simulink model "adc"  (R2017a)
settings: Solver=VariableStepAuto  StartTime=0.0  StopTime=0.0021  FixedStep=0.1e-6  RelTol=1e-3
libraries: simulink x3
settings Model: Creator=Andrei Purcarus  LastModifiedBy=Andrei Purcarus

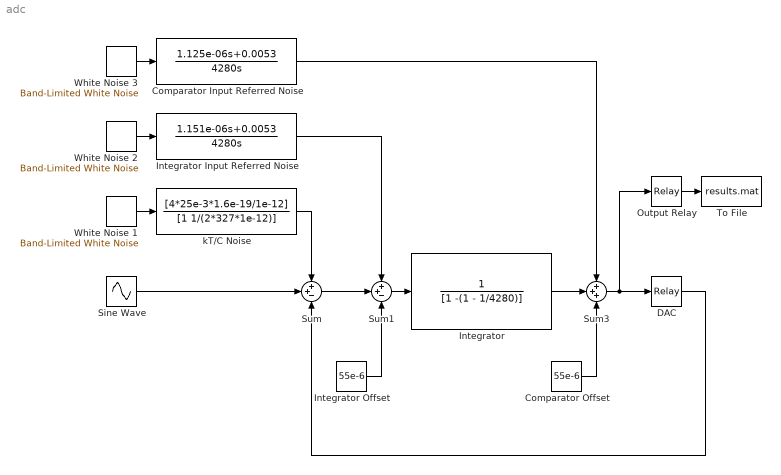
== system adc ==
  Comparator Input Referred Noise : TransferFcn  Numerator=[1.125e-06 0.0053]  Denominator=[4280 0]
  Comparator Offset : Constant  Value=55e-6
  DAC : Relay  OnSwitchValue=0.6  OffSwitchValue=0.6  OnOutputValue=0.6+0.24  OffOutputValue=0.6-0.24
  Integrator : DiscreteTransferFcn  Denominator=[1 -(1 - 1/4280)]  SampleTime=1e-7
  Integrator Input Referred Noise : TransferFcn  Numerator=[1.151e-06 0.0053]  Denominator=[4280 0]
  Integrator Offset : Constant  Value=55e-6
  Output Relay : Relay  OnSwitchValue=0.6  OffSwitchValue=0.6  OnOutputValue=1.2
  Sine Wave : Sin  Amplitude=0.2  Bias=0.6  Frequency=2*pi*20000  SampleTime=0
  Sum : Sum  Inputs=++-
  Sum1 : Sum  Inputs=++-
  Sum3 : Sum  Inputs=+++
  To File : ToFile  Filename=results.mat  SaveFormat=Timeseries  SampleTime=1e-7
  White Noise 1 : simulink/Sources/Band-Limited White Noise  Cov=1  Ts=1e-9  seed=[12343]
  White Noise 2 : simulink/Sources/Band-Limited White Noise  Cov=1  Ts=1e-9  seed=[23341]
  White Noise 3 : simulink/Sources/Band-Limited White Noise  Cov=1  Ts=1e-9  seed=[27231]
  kT/C Noise : TransferFcn  Numerator=[4*25e-3*1.6e-19/1e-12]  Denominator=[1 1/(2*327*1e-12)]
  wires:
  White Noise 2/1 -> Integrator Input Referred Noise/1
  Integrator Input Referred Noise/1 -> Sum1/1
  Sum1/1 -> Integrator/1
  Integrator Offset/1 -> Sum1/3
  Sum3/1 -> Output Relay/1, DAC/1
  Comparator Input Referred Noise/1 -> Sum3/1
  Comparator Offset/1 -> Sum3/3
  White Noise 3/1 -> Comparator Input Referred Noise/1
  Sum/1 -> Sum1/2
  Output Relay/1 -> To File/1
  kT/C Noise/1 -> Sum/1
  White Noise 1/1 -> kT/C Noise/1
  Sine Wave/1 -> Sum/2
  DAC/1 -> Sum/3
  Integrator/1 -> Sum3/2
